simulink model "Battery_pack_recovered"  (R2026b)
settings: Solver=VariableStepAuto  StopTime=12*60*60
settings Model: Creator=yashrajjagtap  LastModifiedBy=yashrajjagtap

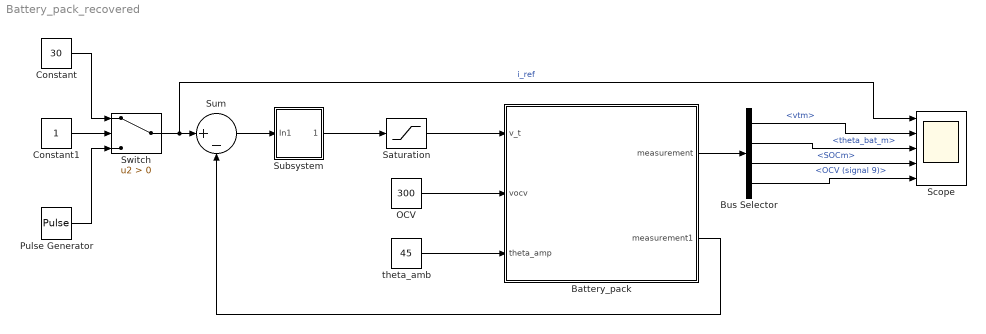
== system Battery_pack_recovered ==
  Battery_pack : Subsystem
  Bus Selector : BusSelector  OutputSignals=m1 (signal 1).vtm,m1 (signal 1).theta_bat_m,m1 (signal 1).SOCm,OCV (signal 9)
  Constant : Constant  Value=30
  Constant1 : Constant
  OCV : Constant  Value=300
  Pulse Generator : DiscretePulseGenerator  PulseType=Time based  Amplitude=15  Period=20*60  PulseWidth=50
  Saturation : Saturate  UpperLimit=320  LowerLimit=0
  Scope : Scope  NumInputPorts=5
      settings: ActiveDisplayYMinimum=20  ActiveDisplayYMaximum=40
  Subsystem : Subsystem
  Sum : Sum  Inputs=|+-
  Switch : Switch  Criteria=u2 > Threshold  SaturateOnIntegerOverflow=off  InputSameDT=off
  theta_amb : Constant  Value=45
  wires:
  Battery_pack/2(measurement1) -> Sum/2
  Sum/1 -> Subsystem/1(In1)
  Subsystem/1(Out1) -> Saturation/1
  Saturation/1 -> Battery_pack/1(v_t)
  OCV/1 -> Battery_pack/2(vocv)
  theta_amb/1 -> Battery_pack/3(theta_amp)
  Battery_pack/1(measurement) -> Bus Selector/1
  Bus Selector/1 -> Scope/2  "<vtm>"
  Bus Selector/2 -> Scope/3  "<theta_bat_m>"
  Bus Selector/3 -> Scope/4  "<SOCm>"
  Switch/1 -> Scope/1, Sum/1  "i_ref"
  Constant/1 -> Switch/1
  Pulse Generator/1 -> Switch/3
  Constant1/1 -> Switch/2
  Bus Selector/4 -> Scope/5  "<OCV (signal 9)>"

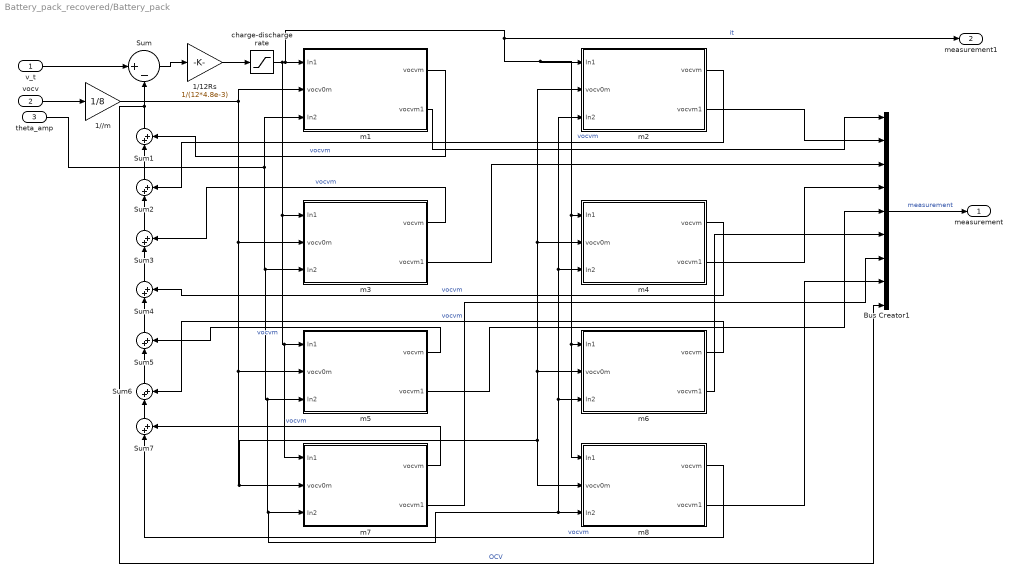
== system Battery_pack_recovered/Battery_pack ==
  v_t : Inport
  vocv : Inport  Port=2
  theta_amp : Inport  Port=3
  1//m : Gain  Gain=1/8
  1/12Rs : Gain  Gain=1/(12*4.8e-3)
  Bus Creator1 : BusCreator  Inputs=9
  Sum : Sum  Inputs=|+-
  Sum{1..7} (7 alike) : Sum  Inputs=|++
  charge-discharge rate : Saturate  UpperLimit=300  LowerLimit=-300
  m1 : Subsystem
  m2 : Subsystem
  m3 : Subsystem
  m4 : Subsystem
  m5 : Subsystem
  m6 : Subsystem
  m7 : Subsystem
  m8 : Subsystem
  measurement : Outport
  measurement1 : Outport  Port=2
  wires:
  m8/2(vocvm1) -> Bus Creator1/8
  m7/2(vocvm1) -> Bus Creator1/7
  m8/1(vocvm) -> Sum7/1  "vocvm"
  m7/1(vocvm) -> Sum7/2  "vocvm"
  m6/1(vocvm) -> Sum6/2  "vocvm"
  Sum4/1 -> Sum3/1
  1//m/1 -> m3/2(vocv0m), m5/2(vocv0m), m7/2(vocv0m), m8/2(vocv0m), m6/2(vocv0m), m4/2(vocv0m), m2/2(vocv0m), m1/2(vocv0m)
  Bus Creator1/1 -> measurement/1  "measurement"
  Sum2/1 -> Sum1/1
  m5/2(vocvm1) -> Bus Creator1/5
  Sum7/1 -> Sum6/1
  m5/1(vocvm) -> Sum5/2  "vocvm"
  m2/2(vocvm1) -> Bus Creator1/2
  vocv/1 -> 1//m/1
  Sum5/1 -> Sum4/1
  Sum/1 -> 1/12Rs/1
  Sum6/1 -> Sum5/1
  m2/1(vocvm) -> Sum2/2  "vocvm"
  m3/2(vocvm1) -> Bus Creator1/3
  Sum1/1 -> Bus Creator1/9, Sum/2  "OCV"
  v_t/1 -> Sum/1
  m6/2(vocvm1) -> Bus Creator1/6
  theta_amp/1 -> m1/3(In2), m3/3(In2), m5/3(In2), m7/3(In2), m8/3(In2), m6/3(In2), m4/3(In2), m2/3(In2)
  m4/1(vocvm) -> Sum4/2  "vocvm"
  m4/2(vocvm1) -> Bus Creator1/4
  m1/2(vocvm1) -> Bus Creator1/1
  m3/1(vocvm) -> Sum3/2  "vocvm"
  m1/1(vocvm) -> Sum1/2  "vocvm"
  Sum3/1 -> Sum2/1
  1/12Rs/1 -> charge-discharge rate/1
  charge-discharge rate/1 -> measurement1/1, m2/1(In1), m4/1(In1), m8/1(In1), m6/1(In1), m1/1(In1), m3/1(In1), m7/1(In1), m5/1(In1)  "it"

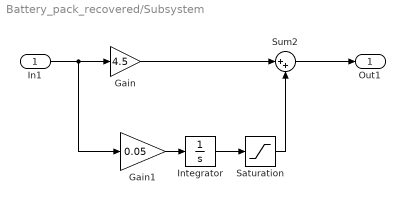
== system Battery_pack_recovered/Subsystem ==
  In1 : Inport
  Gain : Gain  Gain=4.5
  Gain1 : Gain  Gain=0.05
  Integrator : Integrator
  Saturation : Saturate  UpperLimit=350.4  LowerLimit=0
  Sum2 : Sum  Inputs=|++
  Out1 : Outport
  wires:
  Saturation/1 -> Sum2/2
  Integrator/1 -> Saturation/1
  In1/1 -> Gain1/1, Gain/1
  Sum2/1 -> Out1/1
  Gain1/1 -> Integrator/1
  Gain/1 -> Sum2/1

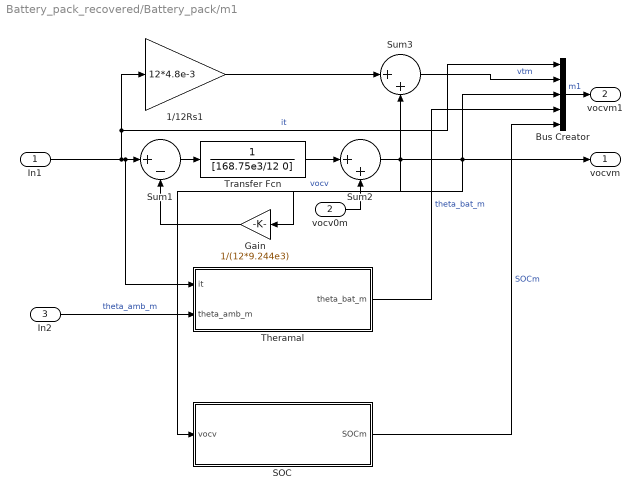
== system Battery_pack_recovered/Battery_pack/m1 ==
  In1 : Inport
  vocv0m : Inport  Port=2
  In2 : Inport  Port=3
  1/12Rs1 : Gain  Gain=12*4.8e-3
  Bus Creator : BusCreator  Inputs=5
  Gain : Gain  Gain=1/(12*9.244e3)
  SOC : Subsystem
  Sum1 : Sum  Inputs=|+-
  Sum2 : Sum  Inputs=|++
  Sum3 : Sum  Inputs=|++
  Theramal : Subsystem
  Transfer Fcn : TransferFcn  Denominator=[168.75e3/12 0]
  vocvm : Outport
  vocvm1 : Outport  Port=2
  wires:
  Sum3/1 -> Bus Creator/2  "vtm"
  Sum1/1 -> Transfer Fcn/1
  Sum2/1 -> Gain/1, Sum3/2, SOC/1(vocv), Bus Creator/3, vocvm/1  "vocv"
  Transfer Fcn/1 -> Sum2/1
  Gain/1 -> Sum1/2
  vocv0m/1 -> Sum2/2
  1/12Rs1/1 -> Sum3/1
  In1/1 -> 1/12Rs1/1, Bus Creator/1, Theramal/1(it), Sum1/1  "it"
  Bus Creator/1 -> vocvm1/1  "m1"
  In2/1 -> Theramal/2(theta_amb_m)  "theta_amb_m"
  Theramal/1(theta_bat_m) -> Bus Creator/4  "theta_bat_m"
  SOC/1(SOCm) -> Bus Creator/5  "SOCm"

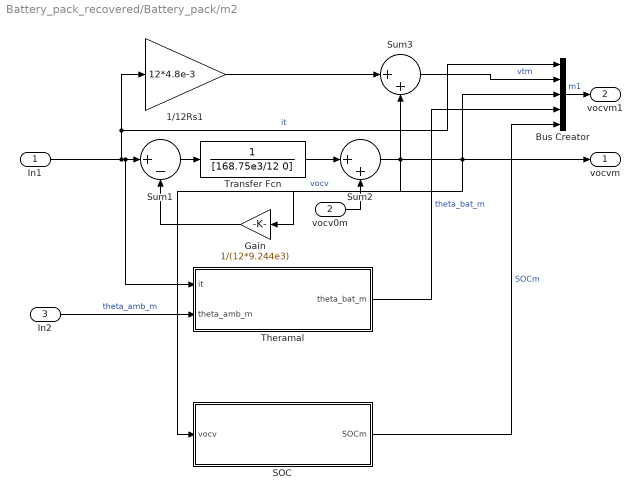
== system Battery_pack_recovered/Battery_pack/m2 ==
  In1 : Inport
  vocv0m : Inport  Port=2
  In2 : Inport  Port=3
  1/12Rs1 : Gain  Gain=12*4.8e-3
  Bus Creator : BusCreator  Inputs=5
  Gain : Gain  Gain=1/(12*9.244e3)
  SOC : Subsystem
  Sum1 : Sum  Inputs=|+-
  Sum2 : Sum  Inputs=|++
  Sum3 : Sum  Inputs=|++
  Theramal : Subsystem
  Transfer Fcn : TransferFcn  Denominator=[168.75e3/12 0]
  vocvm : Outport
  vocvm1 : Outport  Port=2
  wires:
  SOC/1(SOCm) -> Bus Creator/5  "SOCm"
  Theramal/1(theta_bat_m) -> Bus Creator/4  "theta_bat_m"
  In2/1 -> Theramal/2(theta_amb_m)  "theta_amb_m"
  Bus Creator/1 -> vocvm1/1  "m1"
  In1/1 -> Sum1/1, Theramal/1(it), Bus Creator/1, 1/12Rs1/1  "it"
  1/12Rs1/1 -> Sum3/1
  vocv0m/1 -> Sum2/2
  Gain/1 -> Sum1/2
  Transfer Fcn/1 -> Sum2/1
  Sum2/1 -> vocvm/1, Bus Creator/3, SOC/1(vocv), Sum3/2, Gain/1  "vocv"
  Sum1/1 -> Transfer Fcn/1
  Sum3/1 -> Bus Creator/2  "vtm"

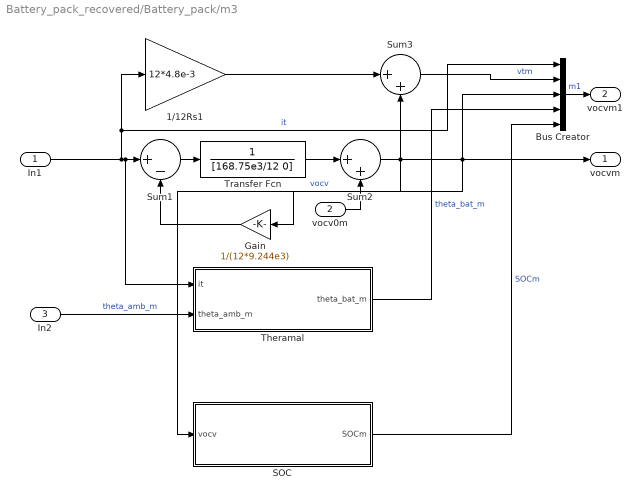
== system Battery_pack_recovered/Battery_pack/m3 ==
  In1 : Inport
  vocv0m : Inport  Port=2
  In2 : Inport  Port=3
  1/12Rs1 : Gain  Gain=12*4.8e-3
  Bus Creator : BusCreator  Inputs=5
  Gain : Gain  Gain=1/(12*9.244e3)
  SOC : Subsystem
  Sum1 : Sum  Inputs=|+-
  Sum2 : Sum  Inputs=|++
  Sum3 : Sum  Inputs=|++
  Theramal : Subsystem
  Transfer Fcn : TransferFcn  Denominator=[168.75e3/12 0]
  vocvm : Outport
  vocvm1 : Outport  Port=2
  wires:
  Sum3/1 -> Bus Creator/2  "vtm"
  Sum1/1 -> Transfer Fcn/1
  Sum2/1 -> Gain/1, Sum3/2, SOC/1(vocv), Bus Creator/3, vocvm/1  "vocv"
  Transfer Fcn/1 -> Sum2/1
  Gain/1 -> Sum1/2
  vocv0m/1 -> Sum2/2
  1/12Rs1/1 -> Sum3/1
  In1/1 -> 1/12Rs1/1, Bus Creator/1, Theramal/1(it), Sum1/1  "it"
  Bus Creator/1 -> vocvm1/1  "m1"
  In2/1 -> Theramal/2(theta_amb_m)  "theta_amb_m"
  Theramal/1(theta_bat_m) -> Bus Creator/4  "theta_bat_m"
  SOC/1(SOCm) -> Bus Creator/5  "SOCm"

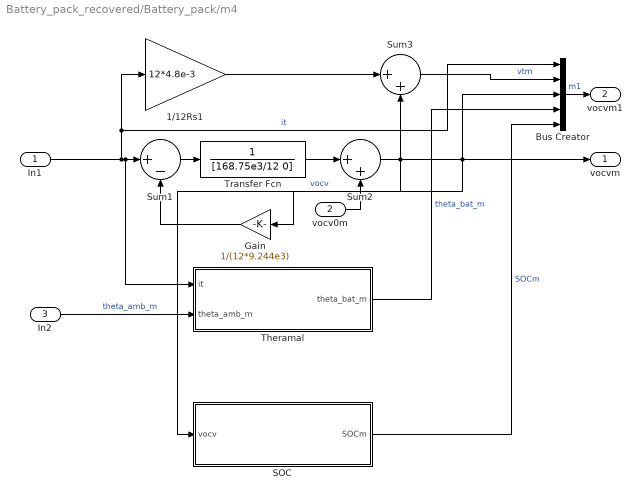
== system Battery_pack_recovered/Battery_pack/m4 ==
  In1 : Inport
  vocv0m : Inport  Port=2
  In2 : Inport  Port=3
  1/12Rs1 : Gain  Gain=12*4.8e-3
  Bus Creator : BusCreator  Inputs=5
  Gain : Gain  Gain=1/(12*9.244e3)
  SOC : Subsystem
  Sum1 : Sum  Inputs=|+-
  Sum2 : Sum  Inputs=|++
  Sum3 : Sum  Inputs=|++
  Theramal : Subsystem
  Transfer Fcn : TransferFcn  Denominator=[168.75e3/12 0]
  vocvm : Outport
  vocvm1 : Outport  Port=2
  wires:
  SOC/1(SOCm) -> Bus Creator/5  "SOCm"
  Theramal/1(theta_bat_m) -> Bus Creator/4  "theta_bat_m"
  In2/1 -> Theramal/2(theta_amb_m)  "theta_amb_m"
  Bus Creator/1 -> vocvm1/1  "m1"
  In1/1 -> Sum1/1, Theramal/1(it), Bus Creator/1, 1/12Rs1/1  "it"
  1/12Rs1/1 -> Sum3/1
  vocv0m/1 -> Sum2/2
  Gain/1 -> Sum1/2
  Transfer Fcn/1 -> Sum2/1
  Sum2/1 -> vocvm/1, Bus Creator/3, SOC/1(vocv), Sum3/2, Gain/1  "vocv"
  Sum1/1 -> Transfer Fcn/1
  Sum3/1 -> Bus Creator/2  "vtm"

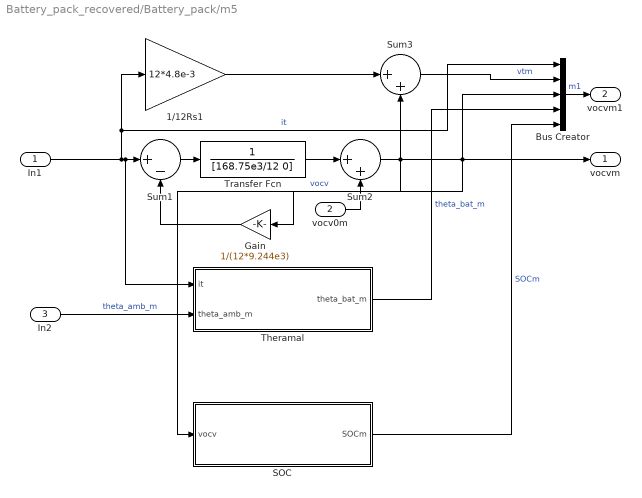
== system Battery_pack_recovered/Battery_pack/m5 ==
  In1 : Inport
  vocv0m : Inport  Port=2
  In2 : Inport  Port=3
  1/12Rs1 : Gain  Gain=12*4.8e-3
  Bus Creator : BusCreator  Inputs=5
  Gain : Gain  Gain=1/(12*9.244e3)
  SOC : Subsystem
  Sum1 : Sum  Inputs=|+-
  Sum2 : Sum  Inputs=|++
  Sum3 : Sum  Inputs=|++
  Theramal : Subsystem
  Transfer Fcn : TransferFcn  Denominator=[168.75e3/12 0]
  vocvm : Outport
  vocvm1 : Outport  Port=2
  wires:
  Sum3/1 -> Bus Creator/2  "vtm"
  Sum1/1 -> Transfer Fcn/1
  Sum2/1 -> Gain/1, Sum3/2, SOC/1(vocv), Bus Creator/3, vocvm/1  "vocv"
  Transfer Fcn/1 -> Sum2/1
  Gain/1 -> Sum1/2
  vocv0m/1 -> Sum2/2
  1/12Rs1/1 -> Sum3/1
  In1/1 -> 1/12Rs1/1, Bus Creator/1, Theramal/1(it), Sum1/1  "it"
  Bus Creator/1 -> vocvm1/1  "m1"
  In2/1 -> Theramal/2(theta_amb_m)  "theta_amb_m"
  Theramal/1(theta_bat_m) -> Bus Creator/4  "theta_bat_m"
  SOC/1(SOCm) -> Bus Creator/5  "SOCm"

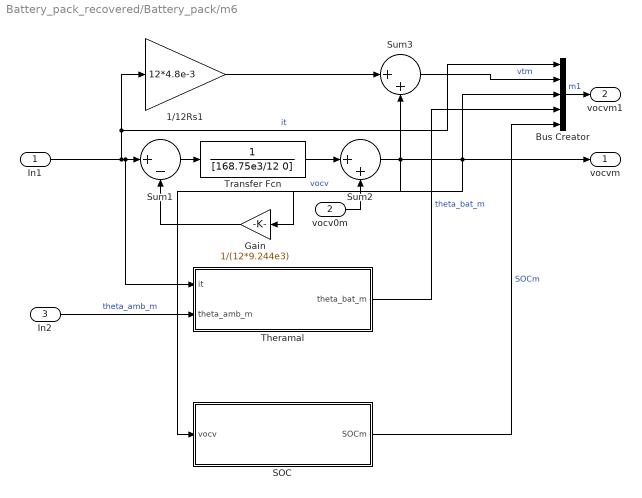
== system Battery_pack_recovered/Battery_pack/m6 ==
  In1 : Inport
  vocv0m : Inport  Port=2
  In2 : Inport  Port=3
  1/12Rs1 : Gain  Gain=12*4.8e-3
  Bus Creator : BusCreator  Inputs=5
  Gain : Gain  Gain=1/(12*9.244e3)
  SOC : Subsystem
  Sum1 : Sum  Inputs=|+-
  Sum2 : Sum  Inputs=|++
  Sum3 : Sum  Inputs=|++
  Theramal : Subsystem
  Transfer Fcn : TransferFcn  Denominator=[168.75e3/12 0]
  vocvm : Outport
  vocvm1 : Outport  Port=2
  wires:
  SOC/1(SOCm) -> Bus Creator/5  "SOCm"
  Theramal/1(theta_bat_m) -> Bus Creator/4  "theta_bat_m"
  In2/1 -> Theramal/2(theta_amb_m)  "theta_amb_m"
  Bus Creator/1 -> vocvm1/1  "m1"
  In1/1 -> Sum1/1, Theramal/1(it), Bus Creator/1, 1/12Rs1/1  "it"
  1/12Rs1/1 -> Sum3/1
  vocv0m/1 -> Sum2/2
  Gain/1 -> Sum1/2
  Transfer Fcn/1 -> Sum2/1
  Sum2/1 -> vocvm/1, Bus Creator/3, SOC/1(vocv), Sum3/2, Gain/1  "vocv"
  Sum1/1 -> Transfer Fcn/1
  Sum3/1 -> Bus Creator/2  "vtm"

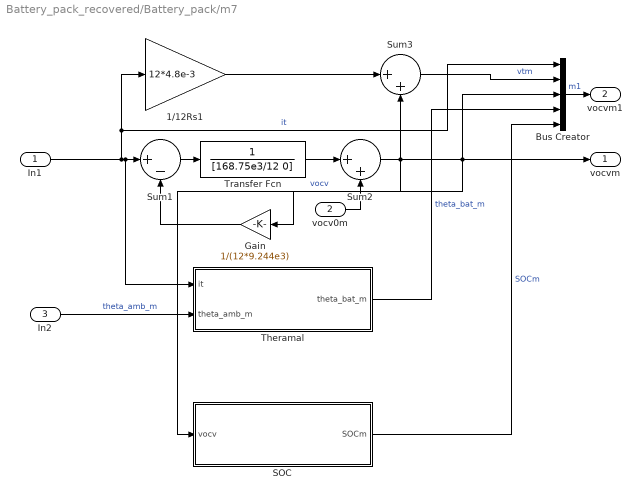
== system Battery_pack_recovered/Battery_pack/m7 ==
  In1 : Inport
  vocv0m : Inport  Port=2
  In2 : Inport  Port=3
  1/12Rs1 : Gain  Gain=12*4.8e-3
  Bus Creator : BusCreator  Inputs=5
  Gain : Gain  Gain=1/(12*9.244e3)
  SOC : Subsystem
  Sum1 : Sum  Inputs=|+-
  Sum2 : Sum  Inputs=|++
  Sum3 : Sum  Inputs=|++
  Theramal : Subsystem
  Transfer Fcn : TransferFcn  Denominator=[168.75e3/12 0]
  vocvm : Outport
  vocvm1 : Outport  Port=2
  wires:
  Sum3/1 -> Bus Creator/2  "vtm"
  Sum1/1 -> Transfer Fcn/1
  Sum2/1 -> Gain/1, Sum3/2, SOC/1(vocv), Bus Creator/3, vocvm/1  "vocv"
  Transfer Fcn/1 -> Sum2/1
  Gain/1 -> Sum1/2
  vocv0m/1 -> Sum2/2
  1/12Rs1/1 -> Sum3/1
  In1/1 -> 1/12Rs1/1, Bus Creator/1, Theramal/1(it), Sum1/1  "it"
  Bus Creator/1 -> vocvm1/1  "m1"
  In2/1 -> Theramal/2(theta_amb_m)  "theta_amb_m"
  Theramal/1(theta_bat_m) -> Bus Creator/4  "theta_bat_m"
  SOC/1(SOCm) -> Bus Creator/5  "SOCm"

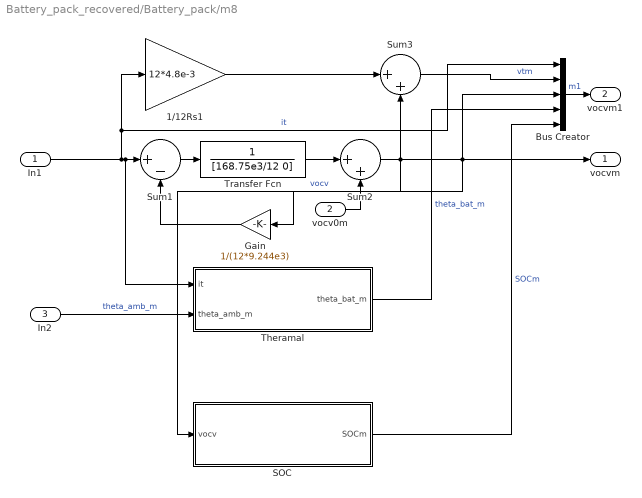
== system Battery_pack_recovered/Battery_pack/m8 ==
  In1 : Inport
  vocv0m : Inport  Port=2
  In2 : Inport  Port=3
  1/12Rs1 : Gain  Gain=12*4.8e-3
  Bus Creator : BusCreator  Inputs=5
  Gain : Gain  Gain=1/(12*9.244e3)
  SOC : Subsystem
  Sum1 : Sum  Inputs=|+-
  Sum2 : Sum  Inputs=|++
  Sum3 : Sum  Inputs=|++
  Theramal : Subsystem
  Transfer Fcn : TransferFcn  Denominator=[168.75e3/12 0]
  vocvm : Outport
  vocvm1 : Outport  Port=2
  wires:
  SOC/1(SOCm) -> Bus Creator/5  "SOCm"
  Theramal/1(theta_bat_m) -> Bus Creator/4  "theta_bat_m"
  In2/1 -> Theramal/2(theta_amb_m)  "theta_amb_m"
  Bus Creator/1 -> vocvm1/1  "m1"
  In1/1 -> Sum1/1, Theramal/1(it), Bus Creator/1, 1/12Rs1/1  "it"
  1/12Rs1/1 -> Sum3/1
  vocv0m/1 -> Sum2/2
  Gain/1 -> Sum1/2
  Transfer Fcn/1 -> Sum2/1
  Sum2/1 -> vocvm/1, Bus Creator/3, SOC/1(vocv), Sum3/2, Gain/1  "vocv"
  Sum1/1 -> Transfer Fcn/1
  Sum3/1 -> Bus Creator/2  "vtm"

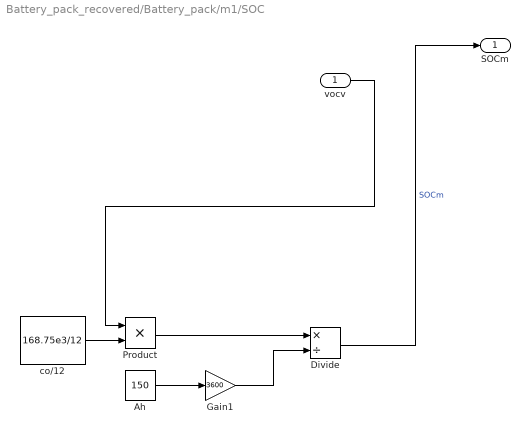
== system Battery_pack_recovered/Battery_pack/m1/SOC ==
  vocv : Inport
  Ah : Constant  Value=150
  Divide : Product  Inputs=*/
  Gain1 : Gain  Gain=3600
  Product : Product
  co/12 : Constant  Value=168.75e3/12
  SOCm : Outport
  wires:
  Gain1/1 -> Divide/2
  Divide/1 -> SOCm/1  "SOCm"
  Product/1 -> Divide/1
  Ah/1 -> Gain1/1
  vocv/1 -> Product/1
  co/12/1 -> Product/2

== system Battery_pack_recovered/Battery_pack/m1/Theramal ==
  it : Inport
  theta_amb_m : Inport  Port=2
  12Rs/mcp : Gain  Gain=12*4.8e-3/(33.792*1020)
  Integrator : Integrator
  Product : Product
  Sum4 : Sum  Inputs=|++
  theta_bat_m : Outport
  wires:
  Sum4/1 -> theta_bat_m/1  "theta_bat_m"
  Integrator/1 -> Sum4/1
  12Rs/mcp/1 -> Integrator/1
  Product/1 -> 12Rs/mcp/1
  theta_amb_m/1 -> Sum4/2
  it/1 -> Product/2, Product/1

== system Battery_pack_recovered/Battery_pack/m2/SOC ==
  vocv : Inport
  Ah : Constant  Value=150
  Divide : Product  Inputs=*/
  Gain1 : Gain  Gain=3600
  Product : Product
  co/12 : Constant  Value=168.75e3/12
  SOCm : Outport
  wires:
  co/12/1 -> Product/2
  vocv/1 -> Product/1
  Ah/1 -> Gain1/1
  Product/1 -> Divide/1
  Divide/1 -> SOCm/1  "SOCm"
  Gain1/1 -> Divide/2

== system Battery_pack_recovered/Battery_pack/m2/Theramal ==
  it : Inport
  theta_amb_m : Inport  Port=2
  12Rs/mcp : Gain  Gain=12*4.8e-3/(33.792*1020)
  Integrator : Integrator
  Product : Product
  Sum4 : Sum  Inputs=|++
  theta_bat_m : Outport
  wires:
  it/1 -> Product/1, Product/2
  theta_amb_m/1 -> Sum4/2
  Product/1 -> 12Rs/mcp/1
  12Rs/mcp/1 -> Integrator/1
  Integrator/1 -> Sum4/1
  Sum4/1 -> theta_bat_m/1  "theta_bat_m"

== system Battery_pack_recovered/Battery_pack/m3/SOC ==
  vocv : Inport
  Ah : Constant  Value=150
  Divide : Product  Inputs=*/
  Gain1 : Gain  Gain=3600
  Product : Product
  co/12 : Constant  Value=168.75e3/12
  SOCm : Outport
  wires:
  Gain1/1 -> Divide/2
  Divide/1 -> SOCm/1  "SOCm"
  Product/1 -> Divide/1
  Ah/1 -> Gain1/1
  vocv/1 -> Product/1
  co/12/1 -> Product/2

== system Battery_pack_recovered/Battery_pack/m3/Theramal ==
  it : Inport
  theta_amb_m : Inport  Port=2
  12Rs/mcp : Gain  Gain=12*4.8e-3/(33.792*1020)
  Integrator : Integrator
  Product : Product
  Sum4 : Sum  Inputs=|++
  theta_bat_m : Outport
  wires:
  Sum4/1 -> theta_bat_m/1  "theta_bat_m"
  Integrator/1 -> Sum4/1
  12Rs/mcp/1 -> Integrator/1
  Product/1 -> 12Rs/mcp/1
  theta_amb_m/1 -> Sum4/2
  it/1 -> Product/2, Product/1

== system Battery_pack_recovered/Battery_pack/m4/SOC ==
  vocv : Inport
  Ah : Constant  Value=150
  Divide : Product  Inputs=*/
  Gain1 : Gain  Gain=3600
  Product : Product
  co/12 : Constant  Value=168.75e3/12
  SOCm : Outport
  wires:
  co/12/1 -> Product/2
  vocv/1 -> Product/1
  Ah/1 -> Gain1/1
  Product/1 -> Divide/1
  Divide/1 -> SOCm/1  "SOCm"
  Gain1/1 -> Divide/2

== system Battery_pack_recovered/Battery_pack/m4/Theramal ==
  it : Inport
  theta_amb_m : Inport  Port=2
  12Rs/mcp : Gain  Gain=12*4.8e-3/(33.792*1020)
  Integrator : Integrator
  Product : Product
  Sum4 : Sum  Inputs=|++
  theta_bat_m : Outport
  wires:
  it/1 -> Product/1, Product/2
  theta_amb_m/1 -> Sum4/2
  Product/1 -> 12Rs/mcp/1
  12Rs/mcp/1 -> Integrator/1
  Integrator/1 -> Sum4/1
  Sum4/1 -> theta_bat_m/1  "theta_bat_m"

== system Battery_pack_recovered/Battery_pack/m5/SOC ==
  vocv : Inport
  Ah : Constant  Value=150
  Divide : Product  Inputs=*/
  Gain1 : Gain  Gain=3600
  Product : Product
  co/12 : Constant  Value=168.75e3/12
  SOCm : Outport
  wires:
  Gain1/1 -> Divide/2
  Divide/1 -> SOCm/1  "SOCm"
  Product/1 -> Divide/1
  Ah/1 -> Gain1/1
  vocv/1 -> Product/1
  co/12/1 -> Product/2

== system Battery_pack_recovered/Battery_pack/m5/Theramal ==
  it : Inport
  theta_amb_m : Inport  Port=2
  12Rs/mcp : Gain  Gain=12*4.8e-3/(33.792*1020)
  Integrator : Integrator
  Product : Product
  Sum4 : Sum  Inputs=|++
  theta_bat_m : Outport
  wires:
  Sum4/1 -> theta_bat_m/1  "theta_bat_m"
  Integrator/1 -> Sum4/1
  12Rs/mcp/1 -> Integrator/1
  Product/1 -> 12Rs/mcp/1
  theta_amb_m/1 -> Sum4/2
  it/1 -> Product/2, Product/1

== system Battery_pack_recovered/Battery_pack/m6/SOC ==
  vocv : Inport
  Ah : Constant  Value=150
  Divide : Product  Inputs=*/
  Gain1 : Gain  Gain=3600
  Product : Product
  co/12 : Constant  Value=168.75e3/12
  SOCm : Outport
  wires:
  co/12/1 -> Product/2
  vocv/1 -> Product/1
  Ah/1 -> Gain1/1
  Product/1 -> Divide/1
  Divide/1 -> SOCm/1  "SOCm"
  Gain1/1 -> Divide/2

== system Battery_pack_recovered/Battery_pack/m6/Theramal ==
  it : Inport
  theta_amb_m : Inport  Port=2
  12Rs/mcp : Gain  Gain=12*4.8e-3/(33.792*1020)
  Integrator : Integrator
  Product : Product
  Sum4 : Sum  Inputs=|++
  theta_bat_m : Outport
  wires:
  it/1 -> Product/1, Product/2
  theta_amb_m/1 -> Sum4/2
  Product/1 -> 12Rs/mcp/1
  12Rs/mcp/1 -> Integrator/1
  Integrator/1 -> Sum4/1
  Sum4/1 -> theta_bat_m/1  "theta_bat_m"

== system Battery_pack_recovered/Battery_pack/m7/SOC ==
  vocv : Inport
  Ah : Constant  Value=150
  Divide : Product  Inputs=*/
  Gain1 : Gain  Gain=3600
  Product : Product
  co/12 : Constant  Value=168.75e3/12
  SOCm : Outport
  wires:
  Gain1/1 -> Divide/2
  Divide/1 -> SOCm/1  "SOCm"
  Product/1 -> Divide/1
  Ah/1 -> Gain1/1
  vocv/1 -> Product/1
  co/12/1 -> Product/2

== system Battery_pack_recovered/Battery_pack/m7/Theramal ==
  it : Inport
  theta_amb_m : Inport  Port=2
  12Rs/mcp : Gain  Gain=12*4.8e-3/(33.792*1020)
  Integrator : Integrator
  Product : Product
  Sum4 : Sum  Inputs=|++
  theta_bat_m : Outport
  wires:
  Sum4/1 -> theta_bat_m/1  "theta_bat_m"
  Integrator/1 -> Sum4/1
  12Rs/mcp/1 -> Integrator/1
  Product/1 -> 12Rs/mcp/1
  theta_amb_m/1 -> Sum4/2
  it/1 -> Product/2, Product/1

== system Battery_pack_recovered/Battery_pack/m8/SOC ==
  vocv : Inport
  Ah : Constant  Value=150
  Divide : Product  Inputs=*/
  Gain1 : Gain  Gain=3600
  Product : Product
  co/12 : Constant  Value=168.75e3/12
  SOCm : Outport
  wires:
  co/12/1 -> Product/2
  vocv/1 -> Product/1
  Ah/1 -> Gain1/1
  Product/1 -> Divide/1
  Divide/1 -> SOCm/1  "SOCm"
  Gain1/1 -> Divide/2

== system Battery_pack_recovered/Battery_pack/m8/Theramal ==
  it : Inport
  theta_amb_m : Inport  Port=2
  12Rs/mcp : Gain  Gain=12*4.8e-3/(33.792*1020)
  Integrator : Integrator
  Product : Product
  Sum4 : Sum  Inputs=|++
  theta_bat_m : Outport
  wires:
  it/1 -> Product/1, Product/2
  theta_amb_m/1 -> Sum4/2
  Product/1 -> 12Rs/mcp/1
  12Rs/mcp/1 -> Integrator/1
  Integrator/1 -> Sum4/1
  Sum4/1 -> theta_bat_m/1  "theta_bat_m"
